simulink model "Expression_EngineSpeed"  (R2020b)
settings: Solver=VariableStepAuto  StartTime=0.0  StopTime=inf  RelTol=1e-3
model workspace (MAT data in the model file):
  x = 1
  y = 0
libraries: simulink x5
settings Model: OrderedModelArguments=off  Creator=dssan  LastModifiedBy=dssan

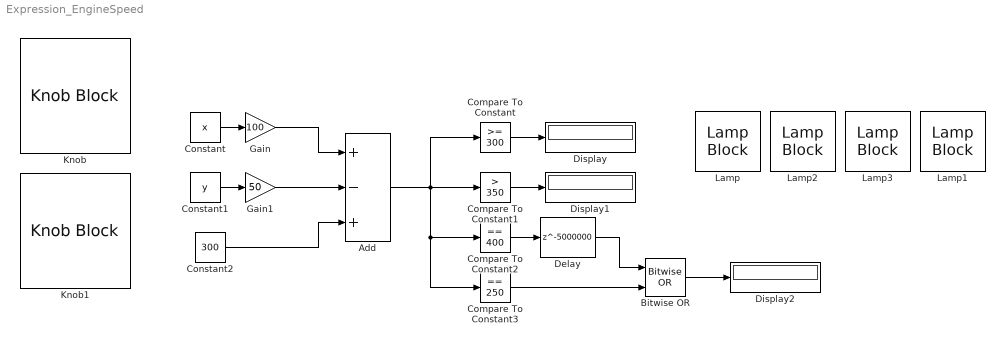
== system Expression_EngineSpeed ==
  Add : Sum  Inputs=+-+
  Bitwise OR : simulink/Logic and Bit Operations/Bitwise Operator  logicop=OR  UseBitMask=off  NumInputPorts=2  BitMask=bin2dec('11011001')  BitMaskRealWorld=Stored Integer
  Compare To Constant : simulink/Logic and Bit Operations/Compare To Constant  relop=>=  const=300  OutDataTypeStr=boolean
  Compare To Constant1 : simulink/Logic and Bit Operations/Compare To Constant  relop=>  const=350  OutDataTypeStr=boolean
  Compare To Constant2 : simulink/Logic and Bit Operations/Compare To Constant  relop===  const=400  OutDataTypeStr=boolean
  Compare To Constant3 : simulink/Logic and Bit Operations/Compare To Constant  relop===  const=250  OutDataTypeStr=boolean
  Constant : Constant  Value=x
  Constant1 : Constant  Value=y
  Constant2 : Constant  Value=300
  Delay : Delay  DelayLength=5000000  InitialCondition=0  UseCircularBuffer=on
  Display : Display
  Display1 : Display
  Display2 : Display
  Gain : Gain  Gain=100
  Gain1 : Gain  Gain=50
  Knob : KnobBlock  ScaleMax=10
  Knob1 : KnobBlock  ScaleMax=10
  Lamp{,1..3} (4 alike) : LampBlock
  wires:
  Gain/1 -> Add/1
  Gain1/1 -> Add/2
  Constant2/1 -> Add/3
  Add/1 -> Compare To Constant3/1, Compare To Constant2/1, Compare To Constant1/1, Compare To Constant/1
  Compare To Constant/1 -> Display/1
  Compare To Constant1/1 -> Display1/1
  Compare To Constant2/1 -> Delay/1
  Compare To Constant3/1 -> Bitwise OR/2
  Constant/1 -> Gain/1
  Constant1/1 -> Gain1/1
  Bitwise OR/1 -> Display2/1
  Delay/1 -> Bitwise OR/1
